simulink model "MLimited"  (R2024b)
settings: configuration reference "STM32H7_Config" (kept outside this file)
settings Model: DataDictionary=Master_Dictionary.sldd  EnableAccessToBaseWorkspace=off  Creator=torni  LastModifiedBy=William
settings ConfigSetRef: SourceName=STM32H7_Config

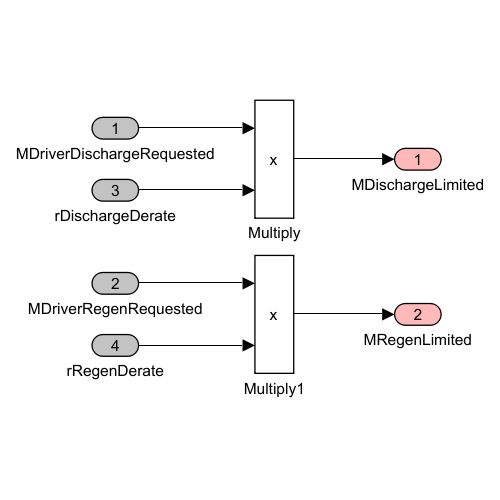
[thumbnail: Simulink's stored preview of the top-level diagram]
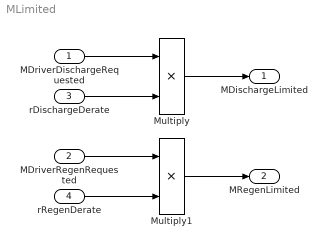
== system MLimited ==
  MDriverDischargeRequested : Inport  OutDataTypeStr=double
  MDriverRegenRequested : Inport  Port=2  OutDataTypeStr=double
  rDischargeDerate : Inport  Port=3  OutDataTypeStr=double
  rRegenDerate : Inport  Port=4  OutDataTypeStr=double
  Multiply : Product
  Multiply1 : Product
  MDischargeLimited : Outport  OutDataTypeStr=double  VectorParamsAs1DForOutWhenUnconnected=off
  MRegenLimited : Outport  Port=2  OutDataTypeStr=double  VectorParamsAs1DForOutWhenUnconnected=off
  wires:
  MDriverDischargeRequested/1 -> Multiply/1
  rDischargeDerate/1 -> Multiply/2
  MDriverRegenRequested/1 -> Multiply1/1
  rRegenDerate/1 -> Multiply1/2
  Multiply/1 -> MDischargeLimited/1
  Multiply1/1 -> MRegenLimited/1
